simulink model "wiper_mdl"  (R2024b)
settings: Solver=FixedStepDiscrete  StartTime=0.0  StopTime=20  FixedStep=0.01  RelTol=1e-3
libraries: simulink x1, SignalEditorBlockLib x1
settings Model: Creator=Hassan Mohamed  LastModifiedBy=Hassan Mohamed

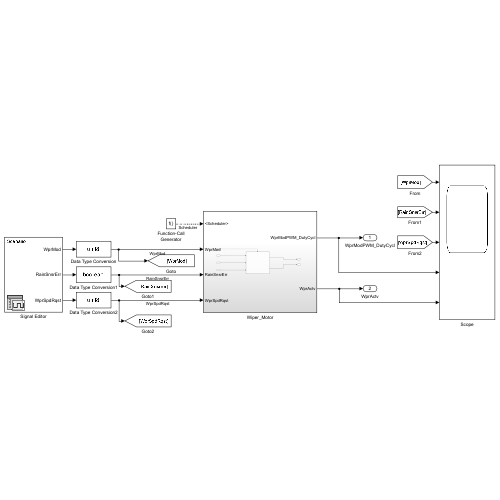
[thumbnail: Simulink's stored preview of the top-level diagram]
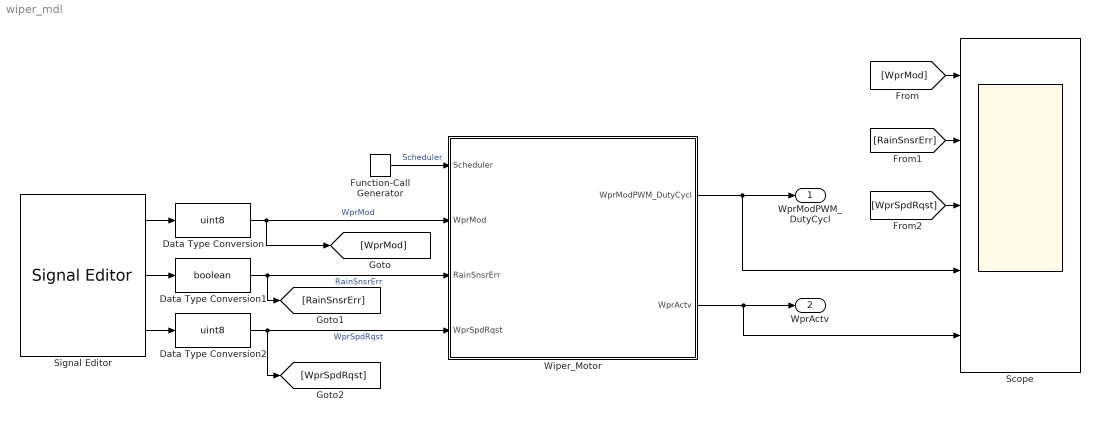
== system wiper_mdl ==
  Data Type Conversion : DataTypeConversion  OutMin=0  OutMax=3  OutDataTypeStr=uint8  SaturateOnIntegerOverflow=off  RndMeth=Floor
  Data Type Conversion1 : DataTypeConversion  OutDataTypeStr=boolean  SaturateOnIntegerOverflow=off  RndMeth=Floor
  Data Type Conversion2 : DataTypeConversion  OutDataTypeStr=uint8  SaturateOnIntegerOverflow=off  RndMeth=Floor
  Function-Call Generator : simulink/Ports & Subsystems/Function-Call Generator  sample_time=1  numberOfIterations=1  DisallowWideOutput=off
  Scope : Scope  NumInputPorts=5
  Signal Editor : SignalEditorBlockLib/Signal Editor  FileName=E:\Automotive\MyPractices\Simulink\WiperSystemControllerSimulink\senario_1.mat  ActiveScenario=Scenario  ActiveSignal=WprMod  IsBus=off  OutputBusObjectStr=Bus: BusObject  SampleTime=0  Interpolate=off  ZeroCross=off  OutputAfterFinalValue=Setting to zero  Unit=inherit  PreserveSignalName=on  ApplySigPropsToAllScenarios=on  ApplySigPropsToAllSignals=on
  Wiper_Motor : Subsystem
  WprModPWM_DutyCycl : Outport
  WprActv : Outport  Port=2
  wires:
  Wiper_Motor/1(WprModPWM_DutyCycl) -> WprModPWM_DutyCycl/1, Scope/4
  Signal Editor/3 -> Data Type Conversion2/1
  Signal Editor/2 -> Data Type Conversion1/1
  Signal Editor/1 -> Data Type Conversion/1
  Wiper_Motor/2(WprActv) -> WprActv/1, Scope/5
  Function-Call Generator/1 -> Wiper_Motor/1(Scheduler)  "Scheduler"
  [RainSnsrErr] -> Scope/2
  [WprMod] -> Scope/1
  [WprSpdRqst] -> Scope/3
  Data Type Conversion/1 -> Wiper_Motor/2(WprMod), [WprMod]  "WprMod"
  Data Type Conversion1/1 -> Wiper_Motor/3(RainSnsrErr), [RainSnsrErr]  "RainSnsrErr"
  Data Type Conversion2/1 -> [WprSpdRqst], Wiper_Motor/4(WprSpdRqst)  "WprSpdRqst"

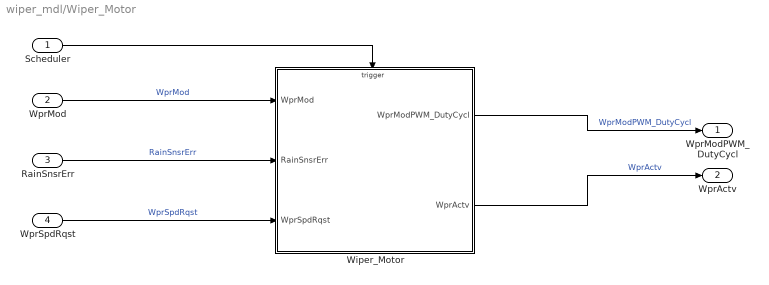
== system wiper_mdl/Wiper_Motor ==
  Scheduler : Inport
  WprMod : Inport  Port=2  OutMin=0  OutMax=3  OutDataTypeStr=uint8
  RainSnsrErr : Inport  Port=3  OutMin=0  OutMax=1  OutDataTypeStr=boolean
  WprSpdRqst : Inport  Port=4  OutMin=0  OutMax=7  OutDataTypeStr=uint8
  Wiper_Motor : Subsystem  TreatAsAtomicUnit=on
  WprModPWM_DutyCycl : Outport
  WprActv : Outport  Port=2
  wires:
  Scheduler/1 -> Wiper_Motor/Trigger
  WprMod/1 -> Wiper_Motor/1(WprMod)  "WprMod"
  RainSnsrErr/1 -> Wiper_Motor/2(RainSnsrErr)  "RainSnsrErr"
  WprSpdRqst/1 -> Wiper_Motor/3(WprSpdRqst)  "WprSpdRqst"
  Wiper_Motor/1(WprModPWM_DutyCycl) -> WprModPWM_DutyCycl/1  "WprModPWM_DutyCycl"
  Wiper_Motor/2(WprActv) -> WprActv/1  "WprActv"

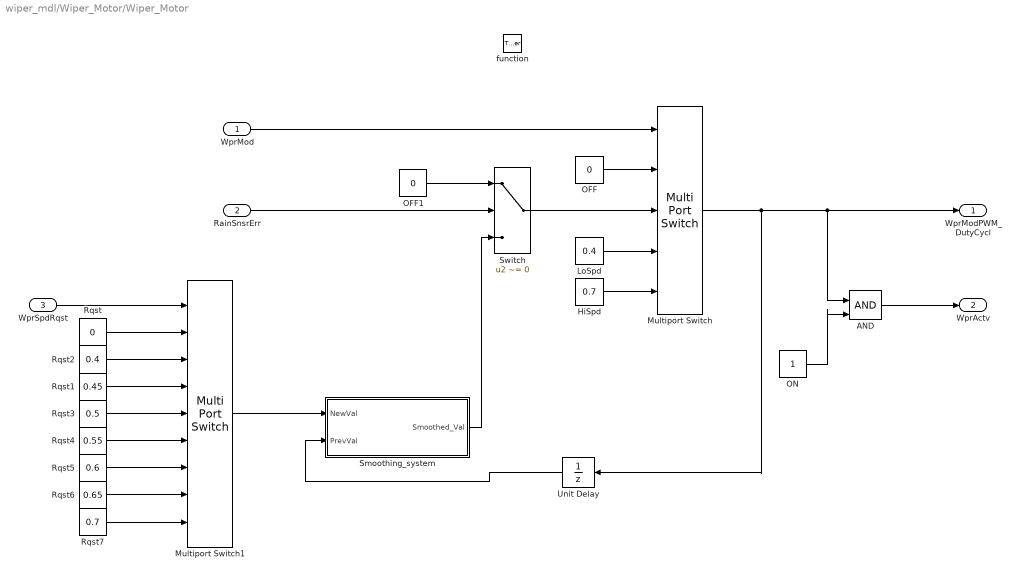
== system wiper_mdl/Wiper_Motor/Wiper_Motor ==
  WprMod : Inport  OutMin=0  OutMax=3  OutDataTypeStr=uint8
  RainSnsrErr : Inport  Port=2  OutMin=0  OutMax=1  OutDataTypeStr=boolean
  WprSpdRqst : Inport  Port=3  OutMin=0  OutMax=7  OutDataTypeStr=uint8
  function : TriggerPort  TriggerType=function-call  VariantControl=(inherit)
  AND : Logic  IconShape=distinctive  AllPortsSameDT=off  OutDataTypeStr=boolean
  HiSpd : Constant  Value=0.7
  LoSpd : Constant  Value=0.4
  Multiport Switch : MultiPortSwitch  DataPortOrder=Zero-based contiguous  Inputs=4  zeroidx=on  OutDataTypeStr=single  SaturateOnIntegerOverflow=off  InputSameDT=off
  Multiport Switch1 : MultiPortSwitch  DataPortOrder=Zero-based contiguous  Inputs=8  zeroidx=on  SaturateOnIntegerOverflow=off  InputSameDT=off
  OFF : Constant  Value=0
  OFF1 : Constant  Value=0
  ON : Constant
  Rqst : Constant  Value=0
  Rqst1 : Constant  Value=0.45
  Rqst2 : Constant  Value=0.4
  Rqst3 : Constant  Value=0.5
  Rqst4 : Constant  Value=0.55
  Rqst5 : Constant  Value=0.6
  Rqst6 : Constant  Value=0.65
  Rqst7 : Constant  Value=0.7
  Smoothing_system : Subsystem  TreatAsAtomicUnit=on
  Switch : Switch  Criteria=u2 ~= 0  SaturateOnIntegerOverflow=off  InputSameDT=off
  Unit Delay : UnitDelay  SampleTime=-1  HasFrameUpgradeWarning=on
  WprModPWM_DutyCycl : Outport
  WprActv : Outport  Port=2
  wires:
  Multiport Switch/1 -> AND/1, WprModPWM_DutyCycl/1, Unit Delay/1
  OFF/1 -> Multiport Switch/2
  LoSpd/1 -> Multiport Switch/4
  HiSpd/1 -> Multiport Switch/5
  Switch/1 -> Multiport Switch/3
  RainSnsrErr/1 -> Switch/2
  OFF1/1 -> Switch/1
  Multiport Switch1/1 -> Smoothing_system/1(NewVal)
  WprSpdRqst/1 -> Multiport Switch1/1
  AND/1 -> WprActv/1
  ON/1 -> AND/2
  Rqst/1 -> Multiport Switch1/2
  Rqst2/1 -> Multiport Switch1/3
  Rqst1/1 -> Multiport Switch1/4
  Rqst3/1 -> Multiport Switch1/5
  Rqst4/1 -> Multiport Switch1/6
  Rqst5/1 -> Multiport Switch1/7
  Rqst6/1 -> Multiport Switch1/8
  Rqst7/1 -> Multiport Switch1/9
  Smoothing_system/1(Smoothed_Val) -> Switch/3
  Unit Delay/1 -> Smoothing_system/2(PrevVal)
  WprMod/1 -> Multiport Switch/1

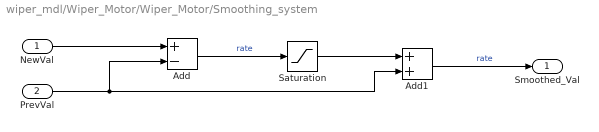
== system wiper_mdl/Wiper_Motor/Wiper_Motor/Smoothing_system ==
  NewVal : Inport
  PrevVal : Inport  Port=2
  Add : Sum  Inputs=+-
  Add1 : Sum
  Saturation : Saturate  UpperLimit=0.01  LowerLimit=-0.01
  Smoothed_Val : Outport
  wires:
  NewVal/1 -> Add/1
  PrevVal/1 -> Add1/2, Add/2
  Add/1 -> Saturation/1  "rate"
  Saturation/1 -> Add1/1
  Add1/1 -> Smoothed_Val/1  "rate"
